simulink model "BLDC_Hysteresis_Control"  (R2025a)
settings: Solver=FixedStepDiscrete  StartTime=0.0  StopTime=1  FixedStep=Ts  RelTol=1e-3  EnableMultiTasking=on
PreLoadFcn:
  | BLDCHysteresisControlData;
undefined symbols (not defined in the file): iref, p, psim, Ts, Tsc, Vdc
libraries: fl_lib x13, nesl_utility x12, ee_lib x4, eeBldcCommutationLogic x1, eeHysteresisControl x1, eeGeneralControl x1
CloseFcn:
  | try,close(h1_BLDCHysteresisControl),end
  | clear h1_BLDCHysteresisControl
  | 
  | clear simlog_BLDCHysteresisControl
  | clear logsout_BLDCHysteresisControl
  | 
  | clear h iref Jm Ls Ms p psim Rs Ts Tsc Vdc
Description:
  | BLDC Hysteresis Current Control
settings Model: Creator=The MathWorks, Inc.  LastModifiedBy=mugun
settings SolverCC: AlgebraicLoopSolver=TrustRegion  MaxZcPerStep=1.0
settings DataIOCC: MaxDataPoints=210000  ReturnWorkspaceOutputs=off  SignalLoggingName=logsout_BLDCHysteresisControl
settings OptimizationCC: ReuseModelBlockBuffer=off  LifeSpan=inf
settings DebuggingCC: UnconnectedInputMsg=warning  UnconnectedOutputMsg=warning  UnconnectedLineMsg=warning  SFUnexpectedBacktrackingDiag=warning  SFNoUnconditionalDefaultTransitionDiag=warning  SFExecutionAtInitializationDiag=none  ArithmeticOperatorsInVariantConditions=warning
settings ModelReferenceCC: EnableRefExpFcnMdlSchedulingChecks=on
settings SFSimCC: SimUseLocalCustomCode=off  CustomCodeUndefinedFunction=UseInterfaceOnly
settings RTWCC: RTWUseLocalCustomCode=off  GPUComputeCapability=3.5  DLArmComputeVersion=19.05
settings CodeAppCC: StateflowObjectComments=on
settings GRTTargetCC: TargetLangStandard=C89/C90 (ANSI)
settings ConfigComp: CovMetricSettings=dw  CovSaveCumulativeToWorkspaceVar=on  CovSaveSingleToWorkspaceVar=on  CovExternalEMLEnable=off
settings SimscapeCC: SimscapeNormalizeSystem=off  SimscapeLogType=all  SimscapeLogSimulationStatistics=on  SimscapeLogName=simlog_BLDCHysteresisControl  SimscapeLogDataHistory=210000.0

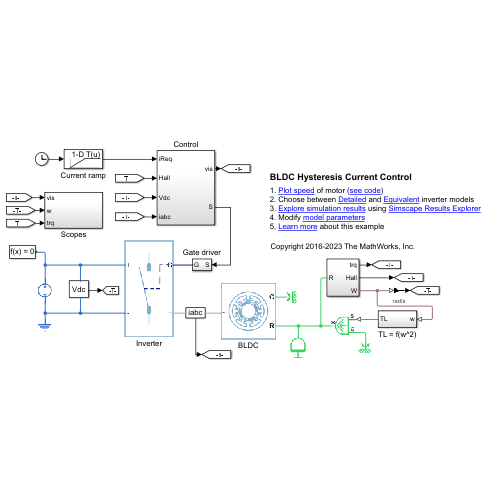
[thumbnail: Simulink's stored preview of the top-level diagram]
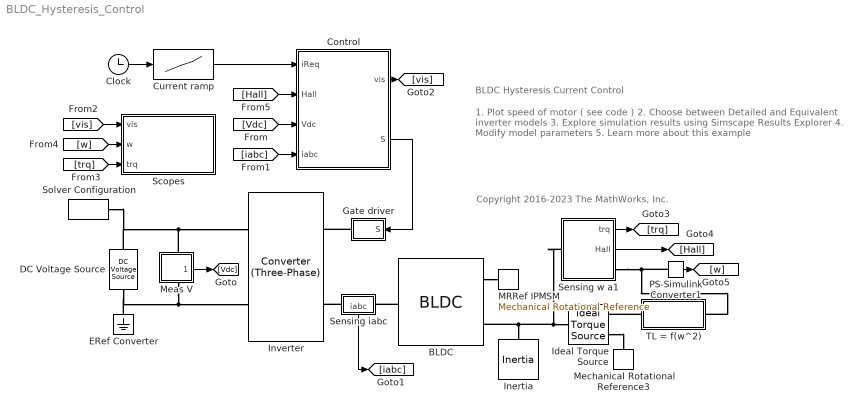
== system BLDC_Hysteresis_Control ==
  note: BLDC Hysteresis Current Control
  note: 1. Plot speed of motor ( see code )
      | 2. Choose between Detailed and Equivalent inverter models
      | 3. Explore simulation results using Simscape Results Explorer
      | 4. Modify model parameters
      | 5. Learn more about this example
  note: Copyright 2016-2023 The MathWorks, Inc.
  BLDC : ee_lib/Electromechanical/Permanent Magnet/BLDC  port_option=ee.enum.threePhasePort.composite  rotor_param=1  pm_flux_linkage=psim Wb  theta_constant=pi / (2*p) rad  emf_max=9.6 V  w_meas=600 rpm  DphiDtheta_tab=[0, -.1528, -.1528, .1528, .1528, 0] Wb/rad  back_emf_tab=[0, -9.6, -9.6, 9.6, 9.6, 0] V  rotor_angle_tab=[0, 7.5, 22.5, 37.5, 52.5, 60] deg  nPolePairs=p  axes_param=1  winding_type=ee.enum.statorconnection.wye  stator_param=2  machine_param=ee.enum.dqparameterization.constant  Ld=0.00022 H  Lq=0.00022 H  idVec=[-200, 0, 200] A  iqVec=[-200, 0, 200] A  LdMatrix=0.00022 * ones(3, 3) H  LqMatrix=0.00022 * ones(3, 3) H  L0=0.00016 H  Ls=Ls H  Lm=0 H  Ms=Ms H  Rs=Rs Ohm  zero_sequence=ee.enum.park.zerosequence.exclude  loss_param=ee.enum.ironloss.none  losses_oc=[0, 0, 0] W  losses_sc=[0, 0, 0] W  f_losses=60 Hz  Isc_losses=95 A  J=0 kg*m^2  lam=0 N*m/(rad/s)  i_d_specify=on  i_d_priority=High  i_d=0 A  i_d_nominal_specify=off  i_d_nominal_value=1  i_d_nominal_unit=A  i_q_specify=on  i_q_priority=High  i_q=0 A  i_q_nominal_specify=off  i_q_nominal_value=1  i_q_nominal_unit=A  torque_specify=off  torque_priority=None  torque=0 N*m  torque_nominal_specify=off  torque_nominal_value=1  torque_nominal_unit=N*m  angular_velocity_specify=off  angular_velocity_priority=High  angular_velocity=0 rpm  angular_velocity_nominal_specify=off  angular_velocity_nominal_value=1  angular_velocity_nominal_unit=rpm  angular_position_specify=off  angular_position_priority=High  angular_position=0 deg  angular_position_nominal_specify=off  angular_position_nominal_value=1  angular_position_nominal_unit=deg  alpha=3.93e-3 1/K  alpha_flux=-0.001 1/K  Tmeas=298.15 K  stator_thermal_mass=100 J/K  rotor_thermal_mass=200 J/K  Rm_percent_rotor=90  Rd_percent_rotor=30  temperatureA_specify=off  temperatureA_priority=High  temperatureA=25 degC  temperatureA_nominal_specify=off  temperatureA_nominal_value=1  temperatureA_nominal_unit=degC  temperatureB_specify=off  temperatureB_priority=High  temperatureB=25 degC  temperatureB_nominal_specify=off  temperatureB_nominal_value=1  temperatureB_nominal_unit=degC  temperatureC_specify=off  temperatureC_priority=High  temperatureC=25 degC  temperatureC_nominal_specify=off  temperatureC_nominal_value=1  temperatureC_nominal_unit=degC  temperatureR_specify=off  temperatureR_priority=High  temperatureR=25 degC  temperatureR_nominal_specify=off  temperatureR_nominal_value=1  temperatureR_nominal_unit=degC
      settings: InternalSimscapePortConfiguration="{\"Bottom\":[],\"Left\":[{\"id\":\"N\",\"label\":\"~\",\"type\":\"foundation.electrical.three_phase\"}],\"Right\":[{\"id\":\"R\",\"label\":\"R\",\"type\":\"foundation.mechanical.rotational.rotational\"},{\"id\":\"C\",\"label\":\"C\",\"type\":\"foundation.mechanical.rotational.rotational\"}],\"Top\":[]}"
  Clock : Clock
  Control : Subsystem
  Current ramp : Lookup_n-D  NumberOfTableDimensions=1  BreakpointsForDimension1=[0 0.5 1]  Table=[0 iref iref]  InternalRulePriority=Speed  RndMeth=Simplest
  DC Voltage Source : fl_lib/Electrical/Electrical Sources/DC Voltage Source  v0=Vdc V
  ERef Converter : fl_lib/Electrical/Electrical Elements/Electrical Reference
  Gate driver : Subsystem
  Ideal Torque Source : fl_lib/Mechanical/Mechanical Sources/Ideal Torque Source
  Inertia : fl_lib/Mechanical/Rotational Elements/Inertia  inertia=Jm kg*m^2  num_ports=foundation.enum.numPorts2.one  w_specify=on  w_priority=High  w=0 rpm  w_nominal_specify=off  w_nominal_value=1  w_nominal_unit=rad/s  t_specify=off  t_priority=High  t=0 N*m  t_nominal_specify=off  t_nominal_value=1  t_nominal_unit=N*m
  Inverter : ee_lib/Semiconductors & Converters/Converters/Converter (Three-Phase)  port_option=ee.enum.threePhasePort.composite  fidelity_option=ee.enum.converters.fidelity.detailed  device_type=3  showThermalPort=false  K=0  Vth=0.5 V  Vgt=1 V  Vgt_off=-1 V  Ih=1 A  Vf=0.8 V  Ron=0.001 Ohm  Rds=0.001 Ohm  Goff=1e-5 1/Ohm  Eon_scalar=22.86e-3 J  Eoff_scalar=17.14e-3 J  Eoff_natural_commutation=10e-3 J  Voff=300 V  Iout_scalar=600 A  onCurrentMeasDelay=0 s  useCurrentFromPreviousCycle=false  useVoltageFromPreviousCycle=false  diode_param=2  diode_Vf=0.8 V  diode_Ron=0.001 Ohm  diode_Goff=1e-5 1/Ohm  diode_C=50 nF  diode_iRM=-235 A  diode_iF=300 A  diode_idot=-50 A/us  diode_trr_param=1  diode_trr_factor=3  diode_trr=15 us  diode_Qrr=1.5e+3 s*uA  diode_rec_loss_model=ee.enum.diode.reverseRecoveryModel.fixed  diode_ErecVal=0 J  diode_scaleWithIandV=false  diode_ErecMat=zeros(2, 3) J  diode_TjrecVec=[298.15, 398.15] K  diode_IfrecVec=[.1, 1, 10] A  diode_IrecVal=10 A  diode_VrecVal=10 V  diode_tFilter=1 / 1000 / 100 s  thermal_network_parameterization=ee.enum.thermalNetworkTopology.external  Rth=[.08, .5] K/W  Rth_Cauer=[.08, .1, .5] K/W  Rth_Foster=[.08, .14, .22, .16] K/W  thermal_mass_parameterization=ee.enum.thermalNetwork.timeconstant  thermal_mass=[.01, .5] J/K  thermal_mass_Cauer=[.01, .1, .5] J/K  thermal_mass_Foster=[.001, .005, .05, .5] J/K  thermal_time_constant=[.001, .2] s  thermal_time_constant_Cauer=[.001, .1, .2] s  thermal_time_constant_Foster=[7e-05, .0007, .01, .08] s  thermal_mass_initial_temperatures=[25, 25] degC  thermal_mass_initial_temperatures_Cauer=[25, 25, 25] degC  junction_thermal_mass=0.01 J/K  Tvec_initial_Foster=[25, 25, 25, 25] degC  snubber_type=0  Cs=1e-7 F  Rs=0.1 Ohm  Vce_loss=[0, 150, 300] V
  MRRef IPMSM : fl_lib/Mechanical/Rotational Elements/Mechanical Rotational Reference
  Meas V : Subsystem
      settings: PortSchema="{\"entries\":[{\"content\":{\"sides\":[{\"content\":{\"connectorIds\":[\"LConn1\"]},\"type\":\"ConnectorPlacement.EquallySpacedRectSide\",\"uuid\":\"9e17bc80-a785-4294-b9db-d48218c93924\"},{\"content\":{\"connectorIds\":[\"RConn1\"],\"side\":\"RIGHT\"},\"type\":\"ConnectorPlacement.EquallySpacedRectSide\",\"uuid\":\"882f999c-bb43-41d5-8f3f-e4b4f1cd965f\"},{\"content\":{\"connectorIds\":[],\"side\":\"TOP\"},\"type\":\"ConnectorPlacement.EquallySpacedRectSide\",\"uuid\":\"0d8306b8-b208-4b52-93ec-7316d462dc74\"},{\"content\":{\"connectorIds\":[\"Out1\"],\"side\":\"BOTTOM\"},\"type\":\"ConnectorPlacement.EquallySpacedRectSide\",\"uuid\":\"375f9460-e008-4114-9f8e-9efcaa8a6b97\"}]},\"type\":\"ConnectorPlacement.EquallySpacedConnector\",\"uuid\":\"d3fdd76d-09cf-465c-b19b-c93af9df2f75\"}],\"packageUris\":[\"http://schema.mathworks.com/mf0/Connector/R2020b\"],\"version\":\"1.0\"}"
      mask Display: disp('Vdc')
  Mechanical Rotational Reference3 : fl_lib/Mechanical/Rotational Elements/Mechanical Rotational Reference
  PS-Simulink Converter1 : nesl_utility/PS-Simulink Converter  PhysicalDomain=network_engine_domain  SubClassName=ps_output  LeftPortType=input  RightPortType=output  PseudoPeriodic=off  Frequencies=[]  VectorFormat=1-D array  Unit=rad/s  AffineConversion=off
  Scopes : Subsystem
  Sensing w a1 : Subsystem
  Sensing iabc : Subsystem
      settings: PortSchema="{\"entries\":[{\"content\":{\"sides\":[{\"content\":{\"connectorIds\":[\"LConn1\"]},\"type\":\"ConnectorPlacement.EquallySpacedRectSide\",\"uuid\":\"d65c841b-b32b-49bd-9628-387529d43346\"},{\"content\":{\"connectorIds\":[\"RConn1\"],\"side\":\"RIGHT\"},\"type\":\"ConnectorPlacement.EquallySpacedRectSide\",\"uuid\":\"6cf26a03-8bd2-4d9d-a8e8-cf9c158ad2d5\"},{\"content\":{\"connectorIds\":[],\"side\":\"TOP\"},\"type\":\"ConnectorPlacement.EquallySpacedRectSide\",\"uuid\":\"233452df-4576-4294-a118-5720dbcd2b4b\"},{\"content\":{\"connectorIds\":[\"Out1\"],\"side\":\"BOTTOM\"},\"type\":\"ConnectorPlacement.EquallySpacedRectSide\",\"uuid\":\"e531e959-bacc-4f25-ab2d-e780a198597e\"}]},\"type\":\"ConnectorPlacement.EquallySpacedConnector\",\"uuid\":\"c5331da1-3503-4f87-b285-4d520d369061\"}],\"packageUris\":[\"http://schema.mathworks.com/mf0/Connector/R2020b\"],\"version\":\"1.0\"}"
      mask Display: disp('iabc')
  Solver Configuration : nesl_utility/Solver Configuration  PhysicalDomain=network_engine_domain  SubClassName=solver  LeftPortType=input  RightPortType=generic  Tones=[]  Harmonics=[]  SimulateNoise=off  Profile=off  UseLocalSampling=off  EnableSwitchedLinearOptims=on  FrequencyDomain=off  UseCCode=off  RelTol=0.001  AbsTol=1e-06  MinStep=1e-09  ToWorkspace=off  RevertToSquareIcSolve=off  NumHomotopyIterations=100  PhasorMode=off  PhasorModeNumHarmonics=1  ConsistencySolver=NEWTON_FTOL  IndexReductionMethod=DerivativeReplacement  DoDC=off  ResidualTolerance=1e-9  ConsistencyTolSource=GLOBAL  ConsistencyAbsTol=0.001  ConsistencyRelTol=0.001  ConsistencyTolFactor=0.001  UseLocalSolver=on  LocalSolverChoice=NE_BACKWARD_EULER_ADVANCER  ResolveIndetEquations=on  FunctionEvalNumThread=1  LocalSolverSampleTime=Ts  DoFixedCost=on  MaxNonlinIter=5  MaxModeIter=2  ComputeImpulses=off  ImpulseIterations=1  LinearAlgebra=auto  LinearAlgebraNumThread=0  EquationFormulation=NE_TIME_EF  DelaysMemoryBudget=1024  AutomaticFiltering=on  FilteringTimeConstant=0.001  PartitionStorageMethod=AS_NEEDED  PartitionMemoryBudget=1024  PartitionMethod=FAST  MultibodyUseLocalSolver=off  MultibodyLocalSolverChoice=ODE1  MultibodyLocalSolverSampleTime=0.001
  TL = f(w^2) : Subsystem
  wires:
  Current ramp/1 -> Control/1(iReq)
  Clock/1 -> Current ramp/1
  [iabc] -> Control/4(iabc)
  [Hall] -> Control/2(Hall)
  [Vdc] -> Control/3(Vdc)
  Control/2(S) -> Gate driver/1(S)
  Meas V/1(vdc) -> [Vdc]
  Sensing iabc/1(iabc) -> [iabc]
  Control/1(vis) -> [vis]
  [vis] -> Scopes/1(vis)
  Sensing w a1/1(trq) -> [trq]
  Sensing w a1/2(Hall) -> [Hall]
  PS-Simulink Converter1/1 -> [w]
  [w] -> Scopes/2(w)
  [trq] -> Scopes/3(trq)
  connections:
  ERef Converter/LConn1 -- DC Voltage Source/RConn1 -- Inverter/RConn2 -- Meas V/RConn1
  Meas V/LConn1 -- Solver Configuration/RConn1 -- DC Voltage Source/LConn1 -- Inverter/RConn1
  Ideal Torque Source/RConn2 -- Mechanical Rotational Reference3/LConn1
  TL = f(w^2)/RConn1 -- Ideal Torque Source/RConn1
  Gate driver/RConn1 -- Inverter/LConn1
  Sensing iabc/LConn1 -- Inverter/LConn2
  Sensing w a1/RConn1 -- PS-Simulink Converter1/LConn1 -- TL = f(w^2)/LConn1
  BLDC/RConn2 -- MRRef IPMSM/LConn1
  Sensing w a1/LConn1 -- BLDC/RConn1 -- Inertia/LConn1 -- Ideal Torque Source/LConn1
  BLDC/LConn1 -- Sensing iabc/RConn1

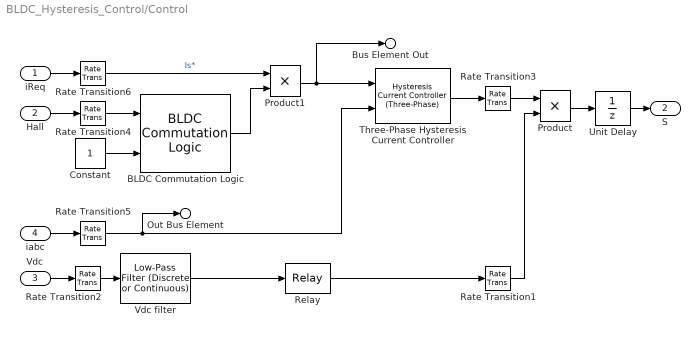
== system BLDC_Hysteresis_Control/Control ==
  iReq : Inport
  Hall : Inport  Port=2
  Vdc : Inport  Port=3
  iabc : Inport  Port=4
  BLDC Commutation Logic : eeBldcCommutationLogic/BLDC Commutation Logic  Ts=Tsc
  Constant : Constant
  Product : Product
  Product1 : Product
  Rate Transition1 : RateTransition  OutPortSampleTime=Ts
  Rate Transition{2,4..6} (4 alike) : RateTransition  OutPortSampleTime=Tsc
  Rate Transition3 : RateTransition  OutPortSampleTime=Ts
  Relay : Relay  OnSwitchValue=Vdc/2  OffSwitchValue=Vdc/4
  Three-Phase Hysteresis Current Controller : eeHysteresisControl/Hysteresis Current Controller (Three-Phase)  h=h  Ts=Tsc
  Unit Delay : UnitDelay  SampleTime=Ts  HasFrameUpgradeWarning=on
  Vdc filter : eeGeneralControl/Low-Pass Filter (Discrete or Continuous)  K=1  T=0.005  B=inf  A=-inf  init_option=Inherited from block input  x0=0  Ts=Tsc
  Bus Element Out : Outport  PortName=vis  Element=iabcRef
  Out Bus Element : Outport  PortName=vis  Element=iabc
  S : Outport  Port=2  VectorParamsAs1DForOutWhenUnconnected=off
  wires:
  Hall/1 -> Rate Transition4/1
  iReq/1 -> Rate Transition6/1
  Rate Transition6/1 -> Product1/1  "Is*"
  Rate Transition4/1 -> BLDC Commutation Logic/1
  BLDC Commutation Logic/1 -> Product1/2
  iabc/1 -> Rate Transition5/1
  Product1/1 -> Bus Element Out/1, Three-Phase Hysteresis Current Controller/1
  Rate Transition5/1 -> Out Bus Element/1, Three-Phase Hysteresis Current Controller/2
  Three-Phase Hysteresis Current Controller/1 -> Rate Transition3/1
  Rate Transition2/1 -> Vdc filter/1
  Vdc filter/1 -> Relay/1
  Vdc/1 -> Rate Transition2/1
  Rate Transition3/1 -> Product/1
  Product/1 -> Unit Delay/1
  Relay/1 -> Rate Transition1/1
  Rate Transition1/1 -> Product/2
  Constant/1 -> BLDC Commutation Logic/2
  Unit Delay/1 -> S/1

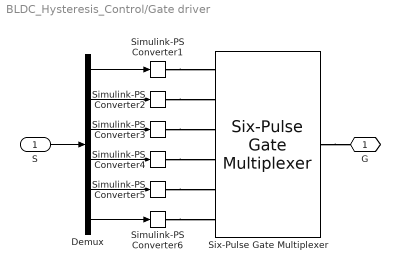
== system BLDC_Hysteresis_Control/Gate driver ==
  S : Inport
  Demux : Demux  Outputs=6
  Simulink-PS Converter{1..6} (6 alike) : nesl_utility/Simulink-PS Converter  PhysicalDomain=network_engine_domain  SubClassName=ps_input  LeftPortType=input  RightPortType=output  PseudoPeriodic=off  Frequencies=[]  NoiseDistribution=none  NoiseParameters=[]  Unit=1  AffineConversion=off  FilteringAndDerivatives=zero  SimscapeFilterOrder=1  InputFilterTimeConstant=0.001  UdotUserProvided=1
  Six-Pulse Gate Multiplexer : ee_lib/Semiconductors & Converters/Converters/Six-Pulse Gate Multiplexer  port_option=ee.enum.controlport.ps
  G : PMIOPort  Side=Right
  wires:
  Demux/1 -> Simulink-PS Converter1/1
  S/1 -> Demux/1
  Demux/4 -> Simulink-PS Converter4/1
  Demux/2 -> Simulink-PS Converter2/1
  Demux/3 -> Simulink-PS Converter3/1
  Demux/5 -> Simulink-PS Converter5/1
  Demux/6 -> Simulink-PS Converter6/1
  connections:
  Six-Pulse Gate Multiplexer/RConn1 -- G/RConn1
  Simulink-PS Converter1/RConn1 -- Six-Pulse Gate Multiplexer/LConn1
  Simulink-PS Converter3/RConn1 -- Six-Pulse Gate Multiplexer/LConn3
  Simulink-PS Converter5/RConn1 -- Six-Pulse Gate Multiplexer/LConn5
  Simulink-PS Converter6/RConn1 -- Six-Pulse Gate Multiplexer/LConn6
  Simulink-PS Converter4/RConn1 -- Six-Pulse Gate Multiplexer/LConn4
  Simulink-PS Converter2/RConn1 -- Six-Pulse Gate Multiplexer/LConn2

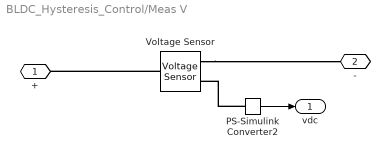
== system BLDC_Hysteresis_Control/Meas V ==
  PS-Simulink Converter2 : nesl_utility/PS-Simulink Converter  PhysicalDomain=network_engine_domain  SubClassName=ps_output  LeftPortType=input  RightPortType=output  PseudoPeriodic=off  Frequencies=[]  VectorFormat=1-D array  Unit=V  AffineConversion=off
  Voltage Sensor : fl_lib/Electrical/Electrical Sensors/Voltage Sensor
  + : PMIOPort  Side=Left
  - : PMIOPort  Port=2  Side=Right
  vdc : Outport
  wires:
  PS-Simulink Converter2/1 -> vdc/1
  connections:
  Voltage Sensor/LConn1 -- +/RConn1
  PS-Simulink Converter2/LConn1 -- Voltage Sensor/RConn1
  Voltage Sensor/RConn2 -- -/RConn1

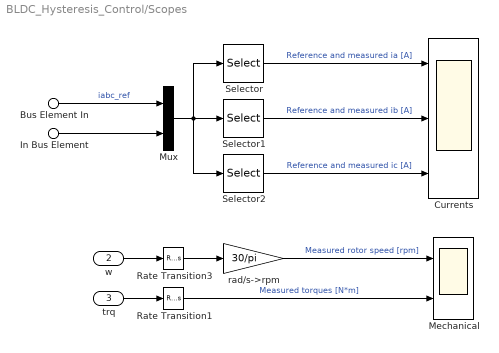
== system BLDC_Hysteresis_Control/Scopes ==
  Bus Element In : Inport  PortName=vis  Element=iabcRef
  In Bus Element : Inport  PortName=vis  Element=iabc
  w : Inport  Port=2
  trq : Inport  Port=3
  Currents : Scope  NumInputPorts=3
      settings: ActiveDisplayYMinimum=-106.65926  ActiveDisplayYMaximum=105.28693
  Mechanical : Scope  NumInputPorts=2
      settings: ActiveDisplayYMinimum=-232.02373  ActiveDisplayYMaximum=1947.99749  DataLoggingVariableName=ScopeData5  DataLoggingSaveFormat=Array
  Mux : Mux  Inputs=2
  Rate Transition1 : RateTransition  OutPortSampleTime=Tsc
  Rate Transition3 : RateTransition  OutPortSampleTime=Tsc
  Selector : Selector  InputPortWidth=6  IndexOptions=Index vector (dialog)  Indices=[1 4]  OutputSizes=1
  Selector1 : Selector  InputPortWidth=6  IndexOptions=Index vector (dialog)  Indices=[2 5]  OutputSizes=1
  Selector2 : Selector  InputPortWidth=6  IndexOptions=Index vector (dialog)  Indices=[3 6]  OutputSizes=1
  rad/s->rpm : Gain  Gain=30/pi
  wires:
  trq/1 -> Rate Transition1/1
  Rate Transition1/1 -> Mechanical/2  "Measured torques [N*m]"
  w/1 -> Rate Transition3/1
  Rate Transition3/1 -> rad/s->rpm/1
  rad/s->rpm/1 -> Mechanical/1  "Measured rotor speed [rpm]"
  Bus Element In/1 -> Mux/1  "iabc_ref"
  In Bus Element/1 -> Mux/2
  Mux/1 -> Selector2/1, Selector1/1, Selector/1
  Selector/1 -> Currents/1  "Reference and measured ia [A]"
  Selector1/1 -> Currents/2  "Reference and measured ib [A]"
  Selector2/1 -> Currents/3  "Reference and measured ic [A]"

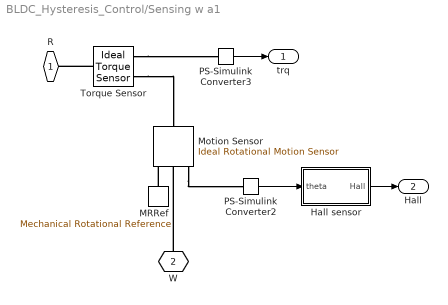
== system BLDC_Hysteresis_Control/Sensing w a1 ==
  Hall sensor : Subsystem
  MRRef : fl_lib/Mechanical/Rotational Elements/Mechanical Rotational Reference
  Motion Sensor : fl_lib/Mechanical/Mechanical Sensors/Ideal Rotational Motion Sensor  reference=foundation.enum.MeasurementReference.difference  acceleration_port=false  velocity_port=true  position_port=true  wrap_angle=simscape.enum.onoff.off  offset=0 deg
  PS-Simulink Converter2 : nesl_utility/PS-Simulink Converter  PhysicalDomain=network_engine_domain  SubClassName=ps_output  LeftPortType=input  RightPortType=output  PseudoPeriodic=off  Frequencies=[]  VectorFormat=1-D array  Unit=rad  AffineConversion=off
  PS-Simulink Converter3 : nesl_utility/PS-Simulink Converter  PhysicalDomain=network_engine_domain  SubClassName=ps_output  LeftPortType=input  RightPortType=output  PseudoPeriodic=off  Frequencies=[]  VectorFormat=1-D array  Unit=N*m  AffineConversion=off
  Torque Sensor : fl_lib/Mechanical/Mechanical Sensors/Ideal Torque Sensor
  R : PMIOPort  Side=Left
  W : PMIOPort  Port=2  Side=Right
  trq : Outport
  Hall : Outport  Port=2
  wires:
  PS-Simulink Converter2/1 -> Hall sensor/1(theta)
  Hall sensor/1(Hall) -> Hall/1
  PS-Simulink Converter3/1 -> trq/1
  connections:
  W/RConn1 -- Motion Sensor/RConn2
  MRRef/LConn1 -- Motion Sensor/RConn1
  Motion Sensor/RConn3 -- PS-Simulink Converter2/LConn1
  Torque Sensor/RConn2 -- PS-Simulink Converter3/LConn1
  Torque Sensor/LConn1 -- R/RConn1
  Torque Sensor/RConn1 -- Motion Sensor/LConn1

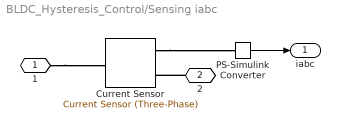
== system BLDC_Hysteresis_Control/Sensing iabc ==
  Current Sensor : ee_lib/Sensors & Transducers/Current Sensor (Three-Phase)
  PS-Simulink Converter : nesl_utility/PS-Simulink Converter  PhysicalDomain=network_engine_domain  SubClassName=ps_output  LeftPortType=input  RightPortType=output  PseudoPeriodic=off  Frequencies=[]  VectorFormat=1-D array  Unit=A  AffineConversion=off
  1 : PMIOPort  Side=Left
  2 : PMIOPort  Port=2  Side=Right
  iabc : Outport
  wires:
  PS-Simulink Converter/1 -> iabc/1
  connections:
  1/RConn1 -- Current Sensor/LConn1
  2/RConn1 -- Current Sensor/RConn2
  Current Sensor/RConn1 -- PS-Simulink Converter/LConn1

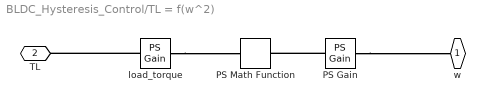
== system BLDC_Hysteresis_Control/TL = f(w^2) ==
  PS Gain : fl_lib/Physical Signals/Functions/PS Gain  gain=1/200 1/(rad/s)
  PS Math Function : fl_lib/Physical Signals/Functions/PS Math Function  fcn_choice=7  v=1
  load_torque : fl_lib/Physical Signals/Functions/PS Gain  gain=-iref*psim*p*1.5 N*m
  w : PMIOPort  Side=Left
  TL : PMIOPort  Port=2  Side=Right
  connections:
  load_torque/RConn1 -- TL/RConn1
  load_torque/LConn1 -- PS Math Function/RConn1
  PS Gain/LConn1 -- w/RConn1
  PS Gain/RConn1 -- PS Math Function/LConn1

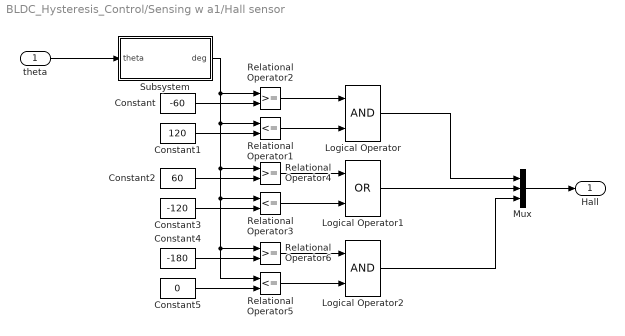
== system BLDC_Hysteresis_Control/Sensing w a1/Hall sensor ==
  theta : Inport
  Constant : Constant  Value=-60
  Constant1 : Constant  Value=120
  Constant2 : Constant  Value=60
  Constant3 : Constant  Value=-120
  Constant4 : Constant  Value=-180
  Constant5 : Constant  Value=0
  Logical Operator : Logic  AllPortsSameDT=off  OutDataTypeStr=boolean
  Logical Operator1 : Logic  Operator=OR  AllPortsSameDT=off  OutDataTypeStr=boolean
  Logical Operator2 : Logic  AllPortsSameDT=off  OutDataTypeStr=boolean
  Mux : Mux  Inputs=3
  Relational Operator1 : RelationalOperator  Operator=<=
  Relational Operator2 : RelationalOperator
  Relational Operator3 : RelationalOperator  Operator=<=
  Relational Operator4 : RelationalOperator
  Relational Operator5 : RelationalOperator  Operator=<=
  Relational Operator6 : RelationalOperator
  Subsystem : Subsystem
  Hall : Outport  VectorParamsAs1DForOutWhenUnconnected=off
  wires:
  Constant3/1 -> Relational Operator3/2
  Logical Operator2/1 -> Mux/3
  Logical Operator1/1 -> Mux/2
  Logical Operator/1 -> Mux/1
  Relational Operator5/1 -> Logical Operator2/2
  Relational Operator6/1 -> Logical Operator2/1
  Constant4/1 -> Relational Operator6/2
  Constant5/1 -> Relational Operator5/2
  Relational Operator3/1 -> Logical Operator1/2
  Mux/1 -> Hall/1
  Relational Operator2/1 -> Logical Operator/1
  Relational Operator1/1 -> Logical Operator/2
  Subsystem/1(deg) -> Relational Operator4/1, Relational Operator3/1, Relational Operator5/1, Relational Operator6/1, Relational Operator1/1, Relational Operator2/1
  Constant/1 -> Relational Operator2/2
  Relational Operator4/1 -> Logical Operator1/1
  Constant1/1 -> Relational Operator1/2
  Constant2/1 -> Relational Operator4/2
  theta/1 -> Subsystem/1(theta)

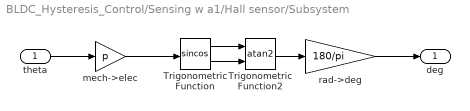
== system BLDC_Hysteresis_Control/Sensing w a1/Hall sensor/Subsystem ==
  theta : Inport
  Trigonometric Function : Trigonometry  Operator=sincos
  Trigonometric Function2 : Trigonometry  Operator=atan2
  mech->elec : Gain  Gain=p
  rad->deg : Gain  Gain=180/pi  SaturateOnIntegerOverflow=on  OutDataTypeStr=Inherit: Same as input  ParamDataTypeStr=Inherit: Same as input
  deg : Outport  VectorParamsAs1DForOutWhenUnconnected=off
  wires:
  Trigonometric Function2/1 -> rad->deg/1
  Trigonometric Function/1 -> Trigonometric Function2/1
  theta/1 -> mech->elec/1
  rad->deg/1 -> deg/1
  Trigonometric Function/2 -> Trigonometric Function2/2
  mech->elec/1 -> Trigonometric Function/1
